simulink model "BMS_EstimateSOC_COM"  (R2022b)
settings: configuration reference "BMS_Sw_CodeGenConfig" (kept outside this file)
model workspace: external: MAT-File H:\0\New MAAM\10 - MBD\Battary Management System\SWE.3 CDD\DataTypes\Data_Script.mat (data not in the file)
undefined symbols (not defined in the file): BATT, DiscIntNeverNeededParam, Schedule
libraries: simulink x4
settings Model: DataDictionary=BMS_Arch_DD.sldd  Creator=MAAM  LastModifiedBy=MAAM
settings ConfigSetRef: SourceName=BMS_Sw_CodeGenConfig

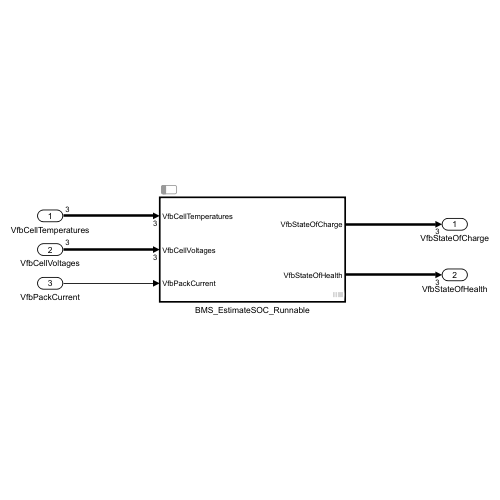
[thumbnail: Simulink's stored preview of the top-level diagram]
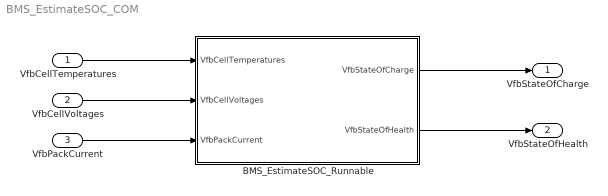
== system BMS_EstimateSOC_COM ==
  VfbCellTemperatures : Inport  OutDataTypeStr=single  Unit=°C
  VfbCellVoltages : Inport  Port=2  OutDataTypeStr=single  Unit=V
  VfbPackCurrent : Inport  Port=3  OutDataTypeStr=single  Unit=A  PortDimensions=1
  BMS_EstimateSOC_Runnable : Subsystem  Tag=BMS_EstimateSOC_Task  Priority=3  TreatAsAtomicUnit=on  ScheduleAs=Periodic partition  PartitionName=BMS_EstimateSOC_Task  SystemSampleTime=Schedule.BMS_EstimateSOC_Task
      settings: RTWSystemCode=Nonreusable function  RTWFcnNameOpts=Use subsystem name  FunctionInterfaceSpec=Allow arguments (Optimized)
  VfbStateOfCharge : Outport  OutDataTypeStr=single
  VfbStateOfHealth : Outport  Port=2  OutDataTypeStr=single
  wires:
  BMS_EstimateSOC_Runnable/1(VfbStateOfCharge) -> VfbStateOfCharge/1
  VfbCellTemperatures/1 -> BMS_EstimateSOC_Runnable/1(VfbCellTemperatures)
  VfbCellVoltages/1 -> BMS_EstimateSOC_Runnable/2(VfbCellVoltages)
  VfbPackCurrent/1 -> BMS_EstimateSOC_Runnable/3(VfbPackCurrent)
  BMS_EstimateSOC_Runnable/2(VfbStateOfHealth) -> VfbStateOfHealth/1

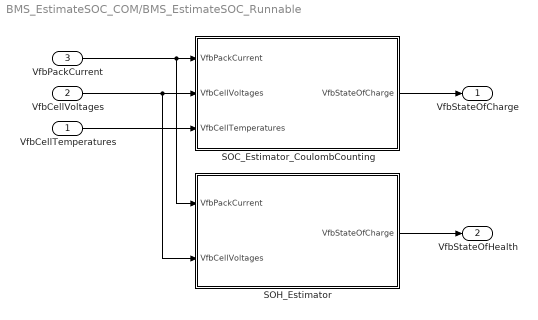
== system BMS_EstimateSOC_COM/BMS_EstimateSOC_Runnable ==
  VfbCellTemperatures : Inport  PortDimensions=BATT.Package.NumModules
  VfbCellVoltages : Inport  Port=2  PortDimensions=BATT.Package.NumModules
  VfbPackCurrent : Inport  Port=3
  SOC_Estimator_CoulombCounting : Subsystem  TreatAsAtomicUnit=on
      settings: RTWSystemCode=Nonreusable function  FunctionInterfaceSpec=Allow arguments (Optimized)
  SOH_Estimator : Subsystem  TreatAsAtomicUnit=on
      settings: RTWSystemCode=Nonreusable function  FunctionInterfaceSpec=Allow arguments (Optimized)
  VfbStateOfCharge : Outport
  VfbStateOfHealth : Outport  Port=2
  wires:
  VfbPackCurrent/1 -> SOH_Estimator/1(VfbPackCurrent), SOC_Estimator_CoulombCounting/1(VfbPackCurrent)
  VfbCellVoltages/1 -> SOH_Estimator/2(VfbCellVoltages), SOC_Estimator_CoulombCounting/2(VfbCellVoltages)
  VfbCellTemperatures/1 -> SOC_Estimator_CoulombCounting/3(VfbCellTemperatures)
  SOC_Estimator_CoulombCounting/1(VfbStateOfCharge) -> VfbStateOfCharge/1
  SOH_Estimator/1(VfbStateOfCharge) -> VfbStateOfHealth/1

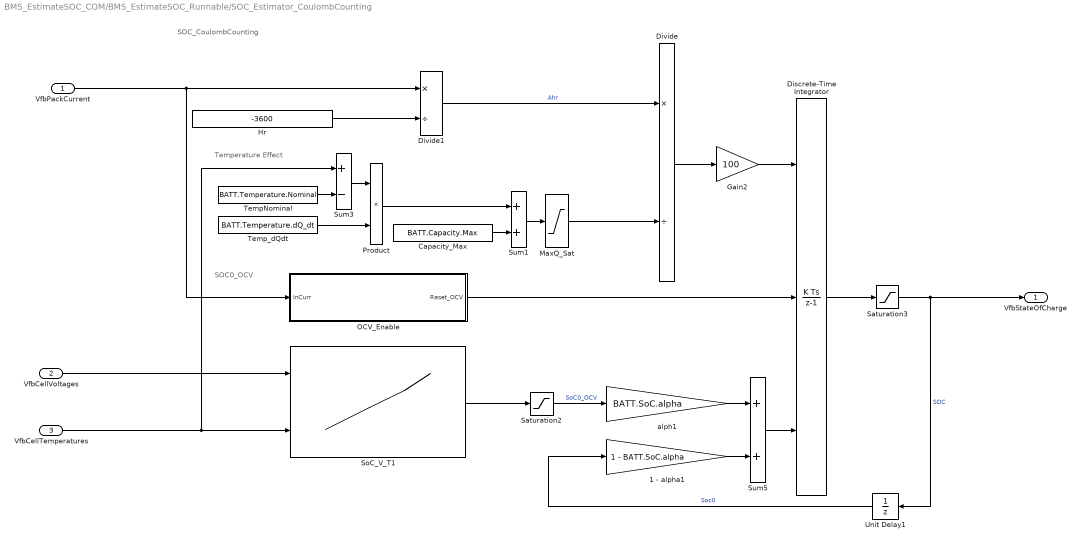
== system BMS_EstimateSOC_COM/BMS_EstimateSOC_Runnable/SOC_Estimator_CoulombCounting ==
  note: SOC_CoulombCounting
  note: Temperature Effect
  note: SOC0_OCV
  VfbPackCurrent : Inport
  VfbCellVoltages : Inport  Port=2  PortDimensions=BATT.Package.NumModules
  VfbCellTemperatures : Inport  Port=3
  1 - alpha1 : Gain  Gain=1 - BATT.SoC.alpha
  Capacity_Max : Constant  Value=BATT.Capacity.Max
  Discrete-Time Integrator : DiscreteIntegrator  ExternalReset=rising  InitialConditionSource=external  InitialCondition=BATT.SOC.SoC0  SampleTime=-1  ICPrevOutput=DiscIntNeverNeededParam  ICPrevScaledInput=DiscIntNeverNeededParam
  Divide : Product  Inputs=*/  OutDataTypeStr=single
  Divide1 : Product  Inputs=*/
  Gain2 : Gain  Gain=100  OutDataTypeStr=single
  Hr : Constant  Value=-3600  OutDataTypeStr=single
  MaxQ_Sat : Saturate  UpperLimit=BATT.Capacity.Max  LowerLimit=0
  OCV_Enable : Subsystem
  Product : Product
  Saturation2 : Saturate  UpperLimit=BATT.SoC.max  LowerLimit=BATT.SoC.min  OutDataTypeStr=single
  Saturation3 : Saturate  UpperLimit=BATT.SoC.max  LowerLimit=BATT.SoC.min  OutDataTypeStr=single
  SoC_V_T1 : Lookup_n-D  BreakpointsForDimension1=BATT.Voltage.V_LUT  BreakpointsForDimension2=BATT.Temperature.T_LUT  Table=BATT.SoC.TableData  InternalRulePriority=Speed  RndMeth=Simplest
      settings: InputPortMap=u0,u1
  Sum1 : Sum
  Sum3 : Sum  Inputs=+-
  Sum5 : Sum
  TempNominal : Constant  Value=BATT.Temperature.Nominal
  Temp_dQdt : Constant  Value=BATT.Temperature.dQ_dt
  Unit Delay1 : UnitDelay  InitialCondition=BATT.SoC.SoC0 * ones(BATT.Package.Ns_Module, BATT.Package.NumModules)  SampleTime=-1  HasFrameUpgradeWarning=on
  alph1 : Gain  Gain=BATT.SoC.alpha
  VfbStateOfCharge : Outport
  wires:
  SoC_V_T1/1 -> Saturation2/1
  Hr/1 -> Divide1/2
  MaxQ_Sat/1 -> Divide/2
  Gain2/1 -> Discrete-Time Integrator/1
  Unit Delay1/1 -> 1 - alpha1/1  "Soc0"
  OCV_Enable/1(Reset_OCV) -> Discrete-Time Integrator/2
  Sum5/1 -> Discrete-Time Integrator/3
  Divide/1 -> Gain2/1
  alph1/1 -> Sum5/1
  1 - alpha1/1 -> Sum5/2
  Discrete-Time Integrator/1 -> Saturation3/1
  Saturation2/1 -> alph1/1  "SoC0_OCV"
  Divide1/1 -> Divide/1  "Ahr"
  Sum1/1 -> MaxQ_Sat/1
  Product/1 -> Sum1/1
  Capacity_Max/1 -> Sum1/2
  Temp_dQdt/1 -> Product/2
  Sum3/1 -> Product/1
  TempNominal/1 -> Sum3/2
  Saturation3/1 -> Unit Delay1/1, VfbStateOfCharge/1  "SOC"
  VfbCellVoltages/1 -> SoC_V_T1/1
  VfbCellTemperatures/1 -> SoC_V_T1/2, Sum3/1
  VfbPackCurrent/1 -> Divide1/1, OCV_Enable/1(InCurr)

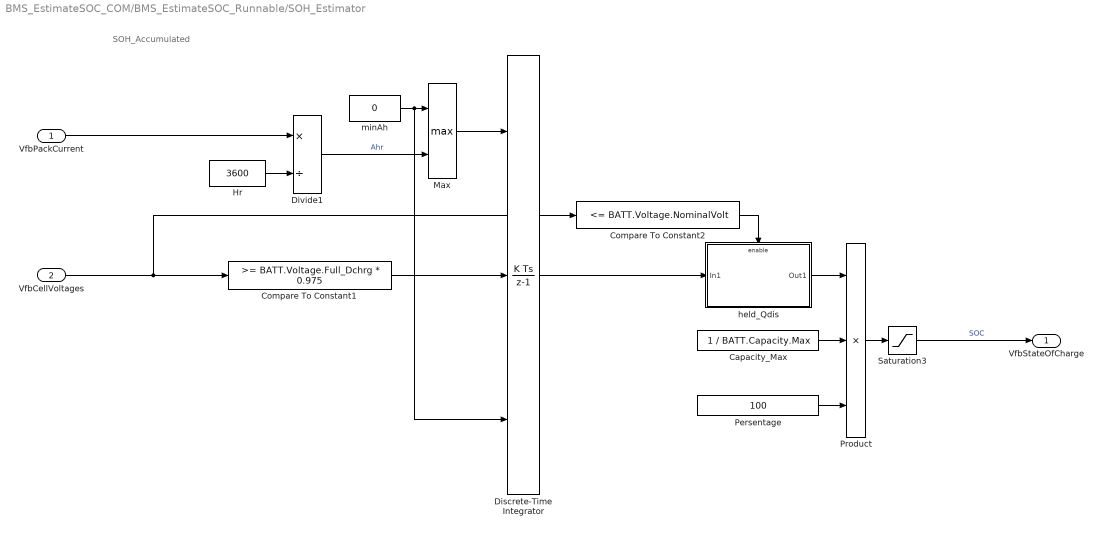
== system BMS_EstimateSOC_COM/BMS_EstimateSOC_Runnable/SOH_Estimator ==
  note: SOH_Accumulated
  VfbPackCurrent : Inport
  VfbCellVoltages : Inport  Port=2  PortDimensions=BATT.Package.NumModules
  Capacity_Max : Constant  Value=1 / BATT.Capacity.Max
  Compare To Constant1 : simulink/Logic and Bit Operations/Compare To Constant  relop=>=  const=BATT.Voltage.Full_Dchrg * 0.975  OutDataTypeStr=boolean
  Compare To Constant2 : simulink/Logic and Bit Operations/Compare To Constant  relop=<=  const=BATT.Voltage.NominalVolt  OutDataTypeStr=boolean
  Discrete-Time Integrator : DiscreteIntegrator  ExternalReset=rising  InitialConditionSource=external  InitialCondition=BATT.SOC.SoC0  SampleTime=-1  ICPrevOutput=DiscIntNeverNeededParam  ICPrevScaledInput=DiscIntNeverNeededParam
  Divide1 : Product  Inputs=*/
  Hr : Constant  Value=3600  OutDataTypeStr=single
  Max : MinMax  Function=max  Inputs=2
  Persentage : Constant  Value=100
  Product : Product  Inputs=3
  Saturation3 : Saturate  UpperLimit=BATT.SoC.max  LowerLimit=BATT.SoC.min  OutDataTypeStr=single
  held_Qdis : Subsystem  TreatAsAtomicUnit=on
  minAh : Constant  Value=0  OutDataTypeStr=single
  VfbStateOfCharge : Outport
  wires:
  VfbPackCurrent/1 -> Divide1/1
  VfbCellVoltages/1 -> Compare To Constant2/1, Compare To Constant1/1
  Saturation3/1 -> VfbStateOfCharge/1  "SOC"
  Divide1/1 -> Max/2  "Ahr"
  Discrete-Time Integrator/1 -> held_Qdis/1(In1)
  Hr/1 -> Divide1/2
  minAh/1 -> Discrete-Time Integrator/3, Max/1
  Max/1 -> Discrete-Time Integrator/1
  Compare To Constant1/1 -> Discrete-Time Integrator/2
  Product/1 -> Saturation3/1
  Compare To Constant2/1 -> held_Qdis/Enable
  held_Qdis/1(Out1) -> Product/1
  Capacity_Max/1 -> Product/2
  Persentage/1 -> Product/3

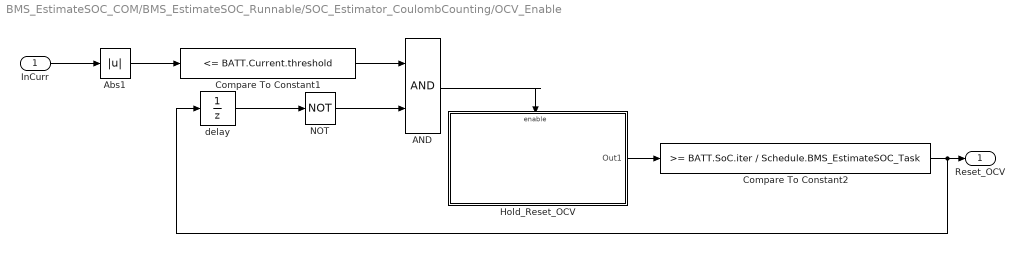
== system BMS_EstimateSOC_COM/BMS_EstimateSOC_Runnable/SOC_Estimator_CoulombCounting/OCV_Enable ==
  InCurr : Inport
  AND : Logic  AllPortsSameDT=off  OutDataTypeStr=boolean
  Abs1 : Abs  SaturateOnIntegerOverflow=off
  Compare To Constant1 : simulink/Logic and Bit Operations/Compare To Constant  relop=<=  const=BATT.Current.threshold  OutDataTypeStr=boolean
  Compare To Constant2 : simulink/Logic and Bit Operations/Compare To Constant  relop=>=  const=BATT.SoC.iter / Schedule.BMS_EstimateSOC_Task  OutDataTypeStr=boolean
  Hold_Reset_OCV : Subsystem
  NOT : Logic  Operator=NOT  AllPortsSameDT=off  OutDataTypeStr=boolean
  delay : UnitDelay  SampleTime=-1  HasFrameUpgradeWarning=on
  Reset_OCV : Outport
  wires:
  InCurr/1 -> Abs1/1
  Compare To Constant1/1 -> AND/1
  Hold_Reset_OCV/1(Out1) -> Compare To Constant2/1
  NOT/1 -> AND/2
  delay/1 -> NOT/1
  AND/1 -> Hold_Reset_OCV/Enable
  Abs1/1 -> Compare To Constant1/1
  Compare To Constant2/1 -> delay/1, Reset_OCV/1

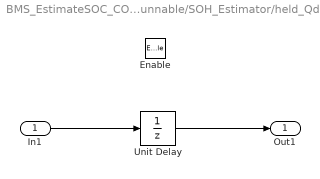
== system BMS_EstimateSOC_COM/BMS_EstimateSOC_Runnable/SOH_Estimator/held_Qdis ==
  In1 : Inport
  Enable : EnablePort
  Unit Delay : UnitDelay  InitialCondition=BATT.Capacity.Max  SampleTime=-1  HasFrameUpgradeWarning=on
  Out1 : Outport
  wires:
  In1/1 -> Unit Delay/1
  Unit Delay/1 -> Out1/1

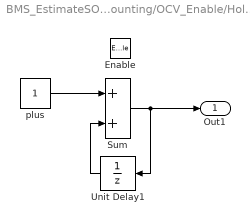
== system BMS_EstimateSOC_COM/BMS_EstimateSOC_Runnable/SOC_Estimator_CoulombCounting/OCV_Enable/Hold_Reset_OCV ==
  Enable : EnablePort  StatesWhenEnabling=reset
  Sum : Sum
  Unit Delay1 : UnitDelay  SampleTime=-1  HasFrameUpgradeWarning=on
  plus : Constant
  Out1 : Outport  OutputWhenDisabled=reset  InitialOutput=0
  wires:
  Unit Delay1/1 -> Sum/2
  Sum/1 -> Out1/1, Unit Delay1/1
  plus/1 -> Sum/1
